simulink model "gm_sampleModel1982_sub"  (R2023a)
settings: Solver=VariableStepAuto  StartTime=0.0  StopTime=10.0  RelTol=1e-3
libraries: hdlsllib x1, simulink x1
settings Model: Creator=user1  LastModifiedBy=user1
settings OptimizationCC: BlockReduction=off  ConditionallyExecuteInputs=off
settings DebuggingCC: InheritedTsInSrcMsg=none

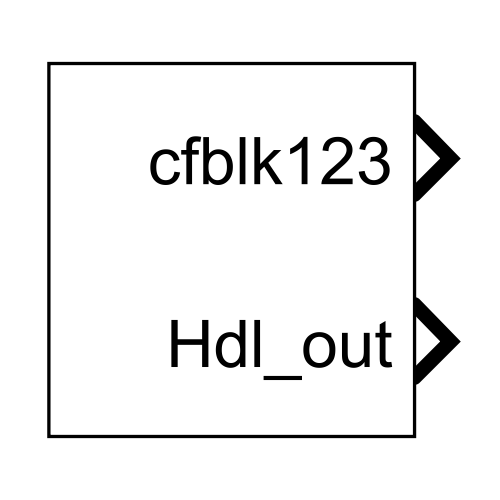
[thumbnail: Simulink's stored preview of the top-level diagram]
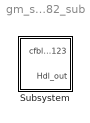
== system gm_sampleModel1982_sub ==
  Subsystem : Subsystem

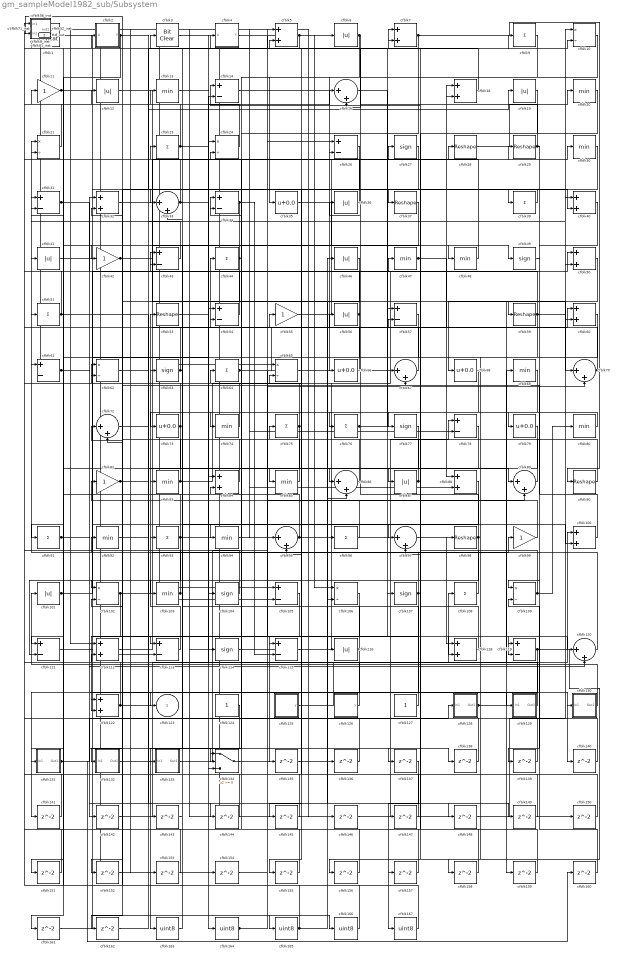
== system gm_sampleModel1982_sub/Subsystem ==
  cfblk1 : hdlsllib/Logic and Bit Operations/Bit Concat  numInputs=2
  cfblk{10,21,24,62,65,102,106,109} (8 alike) : Product  Inputs=*/  OutDataTypeStr=uint8  RndMeth=Zero  SaturateOnIntegerOverflow=on
  cfblk{5,7,18,32,40,50,60,84,88,100,112,118,122} (13 alike) : Sum  OutDataTypeStr=uint8
  cfblk{6,12,19,36,41,46,56,87,101,116} (10 alike) : Abs  OutDataTypeStr=uint8  SaturateOnIntegerOverflow=off
  cfblk{13,20,30,47..48,69,74,80,83,85,92,94,103} (13 alike) : MinMax  OutDataTypeStr=uint8
  cfblk{27,49,63,77,104,107,114} (7 alike) : Signum
  cfblk{14,26,31,34,43,54,57,61,78,105,111,113,115,119} (14 alike) : Sum  Inputs=+-  OutDataTypeStr=uint8
  cfblk{9,23,39,44,51,64,75..76,91,93,96,108} (12 alike) : Sum  Inputs=+  OutDataTypeStr=uint8
  cfblk{11,42,55,82,99} (5 alike) : Gain  OutDataTypeStr=uint8
  cfblk110_inst : Subsystem
  cfblk117_inst : Subsystem
  cfblk{16,33,67,70,72,86,89,95,97,120} (10 alike) : Sum  Inputs=|++  OutDataTypeStr=uint8
  cfblk121_inst : Subsystem
  cfblk124 : Constant  OutDataTypeStr=uint8  SampleTime=-1
  cfblk125 : Subsystem  mask(Counter Free-Running){NumBits=double(16), tsamp=double(-1)}
      mask prompts: NumBits "Simulink:masks:NumberOfBits_MP"; tsamp "Simulink:masks:SampleTime_MP"
      mask help: Simulink:masks:CounterFreeRunning_MD
  cfblk126 : Subsystem  mask(Counter Limited){uplimit=double(7), tsamp=double(-1)}
      mask prompts: uplimit "Simulink:masks:UpperLimit_MP"; tsamp "Simulink:masks:SampleTime_MP"
      mask help: Simulink:masks:CounterLimited_MD
      mask init:
      | nbits = double(8);
      | tsamp = double(-1);
      | uplimit = double(7);
  cfblk127 : Constant  OutDataTypeStr=uint8  SampleTime=-1
  cfblk128 : Subsystem
  cfblk129 : Subsystem
  cfblk130 : Subsystem
  cfblk131 : Subsystem
  cfblk132 : Subsystem
  cfblk133 : Subsystem
  cfblk134 : Switch  OutDataTypeStr=uint8  SaturateOnIntegerOverflow=off  InputSameDT=off
  cfblk{135..162} (28 alike) : Delay  SampleTime=1
  cfblk15_inst : Subsystem
  cfblk{163..167} (5 alike) : DataTypeConversion  OutDataTypeStr=uint8  SaturateOnIntegerOverflow=off  RndMeth=Floor
  cfblk17_inst : Subsystem
  cfblk2 : Subsystem  mask(Detect Fall Nonpositive){vinit=double(0), InputProcessing=Elements as channels (sample based), OutDataTypeStr=uint8}
      mask prompts: vinit "Simulink:masks:InitialCondition_MP"; InputProcessing "Simulink:masks:InputProcessing_MP"; OutDataTypeStr "Simulink:masks:OutputDataType_MP"
      mask help: Simulink:masks:DetectFallNonpositive_MD
      mask init:
      | InputProcessing = 'Elements as channels (sample based)';
      | OutDataTypeStr = 'uint8';
      | vinit = double(0);
      mask TypeOptions InputProcessing: Simulink:masks:ColumnsAsChannelsFrameBased | Simulink:masks:ElementsAsChannelsSampleBased
      mask TypeOptions OutDataTypeStr: Simulink:masks:uint8 | Simulink:masks:boolean
      mask Display: fprintf('U <= 0\n&  NOT\nU/z <= 0')
  cfblk22_inst : Subsystem
  cfblk25_inst : Subsystem
  cfblk{28..29,37,53,59,90,98} (7 alike) : Reshape
  cfblk3 : simulink/Logic and Bit Operations/Bit Clear  iBit=0
      settings: LibrarySourceBlock=|
      | hdlsllib/Logic and Bit
      | Operations/Bit Clear
  cfblk{35,66,68,73,79} (5 alike) : Bias  Bias=0.0  SaturateOnIntegerOverflow=off
  cfblk38_inst : Subsystem
  cfblk4 : Subsystem  mask(Detect Fall Nonpositive){vinit=double(0), InputProcessing=Elements as channels (sample based), OutDataTypeStr=uint8}
      mask prompts: vinit "Simulink:masks:InitialCondition_MP"; InputProcessing "Simulink:masks:InputProcessing_MP"; OutDataTypeStr "Simulink:masks:OutputDataType_MP"
      mask help: Simulink:masks:DetectFallNonpositive_MD
      mask init:
      | InputProcessing = 'Elements as channels (sample based)';
      | OutDataTypeStr = 'uint8';
      | vinit = double(0);
      mask TypeOptions InputProcessing: Simulink:masks:ColumnsAsChannelsFrameBased | Simulink:masks:ElementsAsChannelsSampleBased
      mask TypeOptions OutDataTypeStr: Simulink:masks:uint8 | Simulink:masks:boolean
      mask Display: fprintf('U <= 0\n&  NOT\nU/z <= 0')
  cfblk45_inst : Subsystem
  cfblk52_inst : Subsystem
  cfblk58_inst : Subsystem
  cfblk71_inst : Subsystem
  cfblk81_inst : Subsystem
  cfblk8_inst : Subsystem
  cfblk123 : Outport  OutDataTypeStr=uint8  SampleTime=1  VectorParamsAs1DForOutWhenUnconnected=off
  Hdl_out : Outport  Port=2  OutDataTypeStr=uint8
  wires:
  cfblk1/1 -> cfblk165/1
  cfblk10/1 -> cfblk66/1
  cfblk100/1 -> cfblk121_inst/2(in2)
  cfblk101/1 -> cfblk119/2, cfblk47/1
  cfblk102/1 -> cfblk28/1, cfblk27/1, cfblk122/2, cfblk99/1
  cfblk103/1 -> cfblk53/1, cfblk17_inst/1(in1)
  cfblk104/1 -> cfblk21/1
  cfblk105/1 -> cfblk122/1
  cfblk106/1 -> cfblk135/1
  cfblk107/1 -> cfblk61/1, cfblk115/1, cfblk132/1(In1)
  cfblk108/1 -> cfblk14/1
  cfblk109/1 -> cfblk55/1, cfblk80/1
  cfblk11/1 -> cfblk39/1, cfblk94/1
  cfblk110_inst/1(out1) -> cfblk113/2, cfblk105/1
  cfblk111/1 -> cfblk140/1
  cfblk112/1 -> cfblk44/1
  cfblk113/1 -> cfblk93/1
  cfblk114/1 -> cfblk30/1
  cfblk115/1 -> cfblk10/1
  cfblk116/1 -> cfblk63/1, cfblk141/1
  cfblk117_inst/1(out1) -> cfblk61/2, cfblk136/1
  cfblk118/1 -> cfblk7/1
  cfblk119/1 -> cfblk156/1, cfblk155/1
  cfblk12/1 -> cfblk129/1(In1)
  cfblk120/1 -> cfblk92/1
  cfblk121_inst/1(out1) -> cfblk116/1
  cfblk122/1 -> cfblk14/2, cfblk21/2, cfblk69/1
  cfblk124/1 -> cfblk163/1
  cfblk125/1(y) -> cfblk100/1
  cfblk126/1(y) -> cfblk64/1
  cfblk127/1 -> cfblk83/1
  cfblk128/1(Out1) -> cfblk159/1, cfblk130/1(In1)
  cfblk129/1(Out1) -> cfblk38_inst/1(in1)
  cfblk13/1 -> cfblk120/1
  cfblk130/1(Out1) -> cfblk101/1
  cfblk131/1(Out1) -> cfblk160/1, cfblk128/1(In1)
  cfblk132/1(Out1) -> cfblk108/1
  cfblk133/1(Out1) -> cfblk5/1
  cfblk134/1 -> cfblk50/1
  cfblk135/1 -> cfblk65/2
  cfblk136/1 -> cfblk112/2
  cfblk137/1 -> cfblk167/1
  cfblk138/1 -> cfblk45_inst/1(in1)
  cfblk139/1 -> cfblk62/1
  cfblk14/1 -> cfblk26/2
  cfblk140/1 -> cfblk52_inst/1(in1)
  cfblk141/1 -> cfblk81_inst/1(in1)
  cfblk142/1 -> cfblk86/2
  cfblk143/1 -> cfblk33/2
  cfblk144/1 -> cfblk43/1
  cfblk145/1 -> cfblk54/2
  cfblk146/1 -> cfblk78/1
  cfblk147/1 -> cfblk84/2
  cfblk148/1 -> cfblk50/2
  cfblk149/1 -> cfblk5/2
  cfblk15_inst/1(out1) -> cfblk110_inst/1(in1)
  cfblk150/1 -> cfblk17_inst/2(in2)
  cfblk151/1 -> cfblk22_inst/2(in2)
  cfblk152/1 -> cfblk102/2
  cfblk153/1 -> cfblk32/2
  cfblk154/1 -> cfblk89/2
  cfblk155/1 -> cfblk8_inst/2(in2)
  cfblk156/1 -> cfblk24/2
  cfblk157/1 -> cfblk34/1
  cfblk158/1 -> cfblk72/1
  cfblk159/1 -> cfblk97/2
  cfblk16/1 -> cfblk107/1
  cfblk160/1 -> cfblk109/2
  cfblk161/1 -> cfblk166/1
  cfblk162/1 -> cfblk7/2
  cfblk163/1 -> cfblk3/1
  cfblk164/1 -> cfblk70/2, cfblk67/2
  cfblk165/1 -> cfblk60/1, cfblk62/2
  cfblk166/1 -> cfblk1/1
  cfblk167/1 -> cfblk1/2
  cfblk17_inst/1(out1) -> cfblk67/1
  cfblk18/1 -> cfblk4/1(U)
  cfblk19/1 -> cfblk97/1
  cfblk2/1(Y) -> cfblk40/2, cfblk91/1
  cfblk20/1 -> cfblk77/1
  cfblk21/1 -> cfblk117_inst/1(in1)
  cfblk22_inst/1(out1) -> cfblk88/2, cfblk105/2, cfblk150/1
  cfblk23/1 -> cfblk59/1, cfblk12/1
  cfblk24/1 -> cfblk81_inst/2(in2)
  cfblk25_inst/1(out1) -> cfblk98/1, cfblk153/1
  cfblk26/1 -> cfblk145/1
  cfblk27/1 -> cfblk37/1
  cfblk28/1 -> cfblk20/1
  cfblk29/1 -> cfblk79/1, cfblk58_inst/1(in1)
  cfblk3/1 -> cfblk164/1
  cfblk30/1 -> cfblk72/2
  cfblk31/1 -> cfblk144/1, cfblk143/1
  cfblk32/1 -> cfblk48/1
  cfblk33/1 -> cfblk45_inst/2(in2), cfblk16/1
  cfblk34/1 -> cfblk73/1, cfblk115/2
  cfblk35/1 -> cfblk49/1
  cfblk36/1 -> cfblk15_inst/1(in1)
  cfblk37/1 -> cfblk161/1
  cfblk38_inst/1(out1) -> cfblk25_inst/2(in2), cfblk154/1
  cfblk39/1 -> cfblk33/1
  cfblk4/1(Y) -> cfblk10/2
  cfblk40/1 -> cfblk139/1
  cfblk41/1 -> cfblk114/1
  cfblk42/1 -> cfblk88/1, cfblk134/3, cfblk96/1
  cfblk43/1 -> cfblk31/1
  cfblk44/1 -> cfblk42/1, cfblk162/1
  cfblk45_inst/1(out1) -> cfblk78/2
  cfblk46/1 -> cfblk133/1(In1)
  cfblk47/1 -> cfblk60/2, cfblk157/1
  cfblk48/1 -> cfblk23/1
  cfblk49/1 -> cfblk109/1
  cfblk5/1 -> cfblk52_inst/2(in2), cfblk106/1
  cfblk50/1 -> cfblk68/1
  cfblk51/1 -> cfblk71_inst/2(in2), cfblk148/1
  cfblk52_inst/1(out1) -> cfblk112/1
  cfblk53/1 -> cfblk104/1
  cfblk54/1 -> cfblk32/1
  cfblk55/1 -> cfblk29/1
  cfblk56/1 -> cfblk22_inst/1(in1), cfblk106/2
  cfblk57/1 -> cfblk151/1
  cfblk58_inst/1(out1) -> cfblk95/1
  cfblk59/1 -> cfblk70/1, cfblk38_inst/2(in2), cfblk111/1
  cfblk6/1 -> cfblk35/1, cfblk16/2, cfblk117_inst/2(in2)
  cfblk60/1 -> cfblk158/1
  cfblk61/1 -> cfblk120/2, cfblk137/1
  cfblk62/1 -> cfblk19/1
  cfblk63/1 -> cfblk43/2, cfblk2/1(U)
  cfblk64/1 -> cfblk18/2, cfblk118/2
  cfblk65/1 -> cfblk46/1
  cfblk66/1 -> cfblk56/1
  cfblk67/1 -> cfblk24/1
  cfblk68/1 -> cfblk103/1
  cfblk69/1 -> cfblk95/2
  cfblk7/1 -> cfblk90/1, cfblk134/2
  cfblk70/1 -> cfblk18/1, cfblk121_inst/1(in1)
  cfblk71_inst/1(out1) -> cfblk147/1, cfblk146/1
  cfblk72/1 -> cfblk86/1
  cfblk73/1 -> cfblk110_inst/2(in2), cfblk131/1(In1)
  cfblk74/1 -> cfblk15_inst/2(in2)
  cfblk75/1 -> cfblk58_inst/2(in2), cfblk102/1
  cfblk76/1 -> cfblk57/1, cfblk119/1
  cfblk77/1 -> cfblk85/1
  cfblk78/1 -> cfblk134/1
  cfblk79/1 -> cfblk87/1
  cfblk8_inst/1(out1) -> cfblk65/1
  cfblk80/1 -> cfblk76/1
  cfblk81_inst/1(out1) -> cfblk6/1
  cfblk82/1 -> cfblk89/1, cfblk40/1
  cfblk83/1 -> cfblk25_inst/1(in1), cfblk100/2, cfblk9/1
  cfblk84/1 -> cfblk11/1
  cfblk85/1 -> cfblk34/2
  cfblk86/1 -> cfblk75/1
  cfblk87/1 -> cfblk41/1, cfblk13/1
  cfblk88/1 -> cfblk113/1
  cfblk89/1 -> cfblk54/1
  cfblk9/1 -> cfblk74/1
  cfblk90/1 -> cfblk8_inst/1(in1)
  cfblk91/1 -> cfblk142/1, cfblk123/1
  cfblk92/1 -> cfblk138/1
  cfblk93/1 -> cfblk57/2, cfblk31/2, cfblk111/2
  cfblk94/1 -> cfblk26/1
  cfblk95/1 -> cfblk149/1, cfblk51/1
  cfblk96/1 -> cfblk84/1
  cfblk97/1 -> cfblk118/1
  cfblk98/1 -> cfblk71_inst/1(in1), cfblk36/1, cfblk152/1
  cfblk99/1 -> cfblk82/1

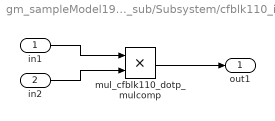
== system gm_sampleModel1982_sub/Subsystem/cfblk110_inst ==
  in1 : Inport  OutDataTypeStr=uint8  SampleTime=1
  in2 : Inport  Port=2  OutDataTypeStr=uint8  SampleTime=1
  mul_cfblk110_dotp_mulcomp : Product  Inputs=**  OutDataTypeStr=uint8  SampleTime=1
  out1 : Outport  OutDataTypeStr=uint8  SampleTime=1
  wires:
  in1/1 -> mul_cfblk110_dotp_mulcomp/1
  in2/1 -> mul_cfblk110_dotp_mulcomp/2
  mul_cfblk110_dotp_mulcomp/1 -> out1/1

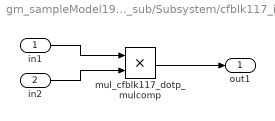
== system gm_sampleModel1982_sub/Subsystem/cfblk117_inst ==
  in1 : Inport  OutDataTypeStr=uint8  SampleTime=1
  in2 : Inport  Port=2  OutDataTypeStr=uint8  SampleTime=1
  mul_cfblk117_dotp_mulcomp : Product  Inputs=**  OutDataTypeStr=uint8  SampleTime=1
  out1 : Outport  OutDataTypeStr=uint8  SampleTime=1
  wires:
  in1/1 -> mul_cfblk117_dotp_mulcomp/1
  in2/1 -> mul_cfblk117_dotp_mulcomp/2
  mul_cfblk117_dotp_mulcomp/1 -> out1/1

== system gm_sampleModel1982_sub/Subsystem/cfblk121_inst ==
  in1 : Inport  OutDataTypeStr=uint8  SampleTime=1
  in2 : Inport  Port=2  OutDataTypeStr=uint8  SampleTime=1
  mul_cfblk121_dotp_mulcomp : Product  Inputs=**  OutDataTypeStr=uint8  SampleTime=1
  out1 : Outport  OutDataTypeStr=uint8  SampleTime=1
  wires:
  in1/1 -> mul_cfblk121_dotp_mulcomp/1
  in2/1 -> mul_cfblk121_dotp_mulcomp/2
  mul_cfblk121_dotp_mulcomp/1 -> out1/1

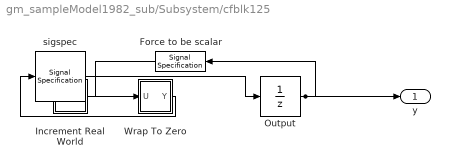
== system gm_sampleModel1982_sub/Subsystem/cfblk125 ==
  Force to be scalar : SignalSpecification  DisableCoverage=on  Dimensions=1
  Increment Real World : Subsystem  mask(Real World Value Increment){}
      mask help: Simulink:masks:RealWorldValueIncrement_MD
      mask Display: disp('V++')
  Output : UnitDelay  InitialCondition=0.0  SampleTime=tsamp  HasFrameUpgradeWarning=on
  Wrap To Zero : Subsystem  mask(Wrap To Zero){Threshold=double(65535)}
      mask prompts: Threshold "Simulink:masks:Threshold_MP"
      mask help: Simulink:masks:WrapToZero_MD
  sigspec : SignalSpecification  OutDataTypeStr=uint16  Dimensions=1
  y : Outport  SampleTime=1
  wires:
  Force to be scalar/1 -> Increment Real World/1(u)
  Increment Real World/1(y) -> Wrap To Zero/1(U)
  Output/1 -> Force to be scalar/1, y/1
  Wrap To Zero/1(Y) -> sigspec/1
  sigspec/1 -> Output/1

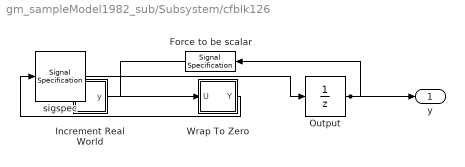
== system gm_sampleModel1982_sub/Subsystem/cfblk126 ==
  Force to be scalar : SignalSpecification  DisableCoverage=on  Dimensions=1
  Increment Real World : Subsystem  mask(Real World Value Increment){}
      mask help: Simulink:masks:RealWorldValueIncrement_MD
      mask Display: disp('V++')
  Output : UnitDelay  InitialCondition=0.0  SampleTime=tsamp  HasFrameUpgradeWarning=on
  Wrap To Zero : Subsystem  mask(Wrap To Zero){Threshold=double(7)}
      mask prompts: Threshold "Simulink:masks:Threshold_MP"
      mask help: Simulink:masks:WrapToZero_MD
  sigspec : SignalSpecification  OutDataTypeStr=uint8  Dimensions=1
  y : Outport  SampleTime=1
  wires:
  Force to be scalar/1 -> Increment Real World/1(u)
  Increment Real World/1(y) -> Wrap To Zero/1(U)
  Output/1 -> Force to be scalar/1, y/1
  Wrap To Zero/1(Y) -> sigspec/1
  sigspec/1 -> Output/1

== system gm_sampleModel1982_sub/Subsystem/cfblk128 ==
  In1 : Inport  OutDataTypeStr=uint8  PortDimensions=1  SampleTime=1
  Out1 : Outport  SampleTime=1
  wires:
  In1/1 -> Out1/1

== system gm_sampleModel1982_sub/Subsystem/cfblk129 ==
  In1 : Inport  OutDataTypeStr=uint8  PortDimensions=1  SampleTime=1
  Out1 : Outport  SampleTime=1
  wires:
  In1/1 -> Out1/1

== system gm_sampleModel1982_sub/Subsystem/cfblk130 ==
  In1 : Inport  OutDataTypeStr=uint8  PortDimensions=1  SampleTime=1
  Out1 : Outport  SampleTime=1
  wires:
  In1/1 -> Out1/1

== system gm_sampleModel1982_sub/Subsystem/cfblk131 ==
  In1 : Inport  OutDataTypeStr=uint8  PortDimensions=1  SampleTime=1
  Out1 : Outport  SampleTime=1
  wires:
  In1/1 -> Out1/1

== system gm_sampleModel1982_sub/Subsystem/cfblk132 ==
  In1 : Inport  OutDataTypeStr=uint8  PortDimensions=1  SampleTime=1
  Out1 : Outport  SampleTime=1
  wires:
  In1/1 -> Out1/1

== system gm_sampleModel1982_sub/Subsystem/cfblk133 ==
  In1 : Inport  OutDataTypeStr=uint8  PortDimensions=1  SampleTime=1
  Out1 : Outport  SampleTime=1
  wires:
  In1/1 -> Out1/1

== system gm_sampleModel1982_sub/Subsystem/cfblk15_inst ==
  in1 : Inport  OutDataTypeStr=uint8  SampleTime=1
  in2 : Inport  Port=2  OutDataTypeStr=uint8  SampleTime=1
  mul_cfblk15_dotp_mulcomp : Product  Inputs=**  OutDataTypeStr=uint8  SampleTime=1
  out1 : Outport  OutDataTypeStr=uint8  SampleTime=1
  wires:
  in1/1 -> mul_cfblk15_dotp_mulcomp/1
  in2/1 -> mul_cfblk15_dotp_mulcomp/2
  mul_cfblk15_dotp_mulcomp/1 -> out1/1

== system gm_sampleModel1982_sub/Subsystem/cfblk17_inst ==
  in1 : Inport  OutDataTypeStr=uint8  SampleTime=1
  in2 : Inport  Port=2  OutDataTypeStr=uint8  SampleTime=1
  mul_cfblk17_dotp_mulcomp : Product  Inputs=**  OutDataTypeStr=uint8  SampleTime=1
  out1 : Outport  OutDataTypeStr=uint8  SampleTime=1
  wires:
  in1/1 -> mul_cfblk17_dotp_mulcomp/1
  in2/1 -> mul_cfblk17_dotp_mulcomp/2
  mul_cfblk17_dotp_mulcomp/1 -> out1/1

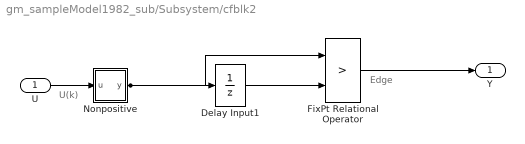
== system gm_sampleModel1982_sub/Subsystem/cfblk2 ==
  note: U(k)
  note: Edge
  U : Inport  OutDataTypeStr=uint8  SampleTime=1
  Delay Input1 : UnitDelay  Description=Store in Global RAM  DisableCoverage=on  InitialCondition=vinit  SampleTime=-1  HasFrameUpgradeWarning=on
  FixPt Relational Operator : RelationalOperator  Operator=>  OutDataTypeStr=fixdt(0, 8)  ZeroCross=off  InputSameDT=off
  Nonpositive : Subsystem  mask(Compare To Zero){relop=<=, OutDataTypeStr=boolean, ZeroCross=off}
      mask prompts: relop "Simulink:masks:Operator_MP"; OutDataTypeStr "Simulink:masks:OutputDataType_MP"; ZeroCross "Simulink:masks:EnableZerocrossingDetection_MP"
      mask help: Simulink:masks:CompareToZero_MD
      mask init:
      | OutDataTypeStr = 'boolean';
      | ZeroCross = 'off';
      | blkName = 'sampleModel1982_sub/Subsystem/cfblk2/Nonpositive';
      | relop = '<=';
      | setValue = 'boolean';
      mask TypeOptions relop: == | ~= | < | <= | >= | >
      mask TypeOptions OutDataTypeStr: Simulink:masks:uint8 | Simulink:masks:boolean
      mask Callback ZeroCross: sl('zeroCrossEnable', gcbh);
      mask Display: disp([relop,' 0'])
  Y : Outport  SampleTime=1
  wires:
  U/1 -> Nonpositive/1(u)
  Delay Input1/1 -> FixPt Relational Operator/2
  FixPt Relational Operator/1 -> Y/1
  Nonpositive/1(y) -> FixPt Relational Operator/1, Delay Input1/1

== system gm_sampleModel1982_sub/Subsystem/cfblk22_inst ==
  in1 : Inport  OutDataTypeStr=uint8  SampleTime=1
  in2 : Inport  Port=2  OutDataTypeStr=uint8  SampleTime=1
  mul_cfblk22_dotp_mulcomp : Product  Inputs=**  OutDataTypeStr=uint8  SampleTime=1
  out1 : Outport  OutDataTypeStr=uint8  SampleTime=1
  wires:
  in1/1 -> mul_cfblk22_dotp_mulcomp/1
  in2/1 -> mul_cfblk22_dotp_mulcomp/2
  mul_cfblk22_dotp_mulcomp/1 -> out1/1

== system gm_sampleModel1982_sub/Subsystem/cfblk25_inst ==
  in1 : Inport  OutDataTypeStr=uint8  SampleTime=1
  in2 : Inport  Port=2  OutDataTypeStr=uint8  SampleTime=1
  mul_cfblk25_dotp_mulcomp : Product  Inputs=**  OutDataTypeStr=uint8  SampleTime=1
  out1 : Outport  OutDataTypeStr=uint8  SampleTime=1
  wires:
  in1/1 -> mul_cfblk25_dotp_mulcomp/1
  in2/1 -> mul_cfblk25_dotp_mulcomp/2
  mul_cfblk25_dotp_mulcomp/1 -> out1/1

== system gm_sampleModel1982_sub/Subsystem/cfblk38_inst ==
  in1 : Inport  OutDataTypeStr=uint8  SampleTime=1
  in2 : Inport  Port=2  OutDataTypeStr=uint8  SampleTime=1
  mul_cfblk38_dotp_mulcomp : Product  Inputs=**  OutDataTypeStr=uint8  SampleTime=1
  out1 : Outport  OutDataTypeStr=uint8  SampleTime=1
  wires:
  in1/1 -> mul_cfblk38_dotp_mulcomp/1
  in2/1 -> mul_cfblk38_dotp_mulcomp/2
  mul_cfblk38_dotp_mulcomp/1 -> out1/1

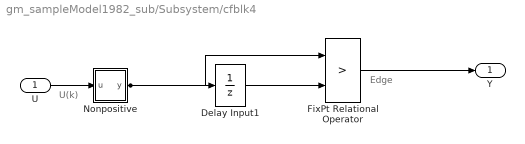
== system gm_sampleModel1982_sub/Subsystem/cfblk4 ==
  note: U(k)
  note: Edge
  U : Inport  OutDataTypeStr=uint8  SampleTime=1
  Delay Input1 : UnitDelay  Description=Store in Global RAM  DisableCoverage=on  InitialCondition=vinit  SampleTime=-1  HasFrameUpgradeWarning=on
  FixPt Relational Operator : RelationalOperator  Operator=>  OutDataTypeStr=fixdt(0, 8)  ZeroCross=off  InputSameDT=off
  Nonpositive : Subsystem  mask(Compare To Zero){relop=<=, OutDataTypeStr=boolean, ZeroCross=off}
      mask prompts: relop "Simulink:masks:Operator_MP"; OutDataTypeStr "Simulink:masks:OutputDataType_MP"; ZeroCross "Simulink:masks:EnableZerocrossingDetection_MP"
      mask help: Simulink:masks:CompareToZero_MD
      mask init:
      | OutDataTypeStr = 'boolean';
      | ZeroCross = 'off';
      | blkName = 'sampleModel1982_sub/Subsystem/cfblk4/Nonpositive';
      | relop = '<=';
      | setValue = 'boolean';
      mask TypeOptions relop: == | ~= | < | <= | >= | >
      mask TypeOptions OutDataTypeStr: Simulink:masks:uint8 | Simulink:masks:boolean
      mask Callback ZeroCross: sl('zeroCrossEnable', gcbh);
      mask Display: disp([relop,' 0'])
  Y : Outport  SampleTime=1
  wires:
  U/1 -> Nonpositive/1(u)
  Delay Input1/1 -> FixPt Relational Operator/2
  FixPt Relational Operator/1 -> Y/1
  Nonpositive/1(y) -> FixPt Relational Operator/1, Delay Input1/1

== system gm_sampleModel1982_sub/Subsystem/cfblk45_inst ==
  in1 : Inport  OutDataTypeStr=uint8  SampleTime=1
  in2 : Inport  Port=2  OutDataTypeStr=uint8  SampleTime=1
  mul_cfblk45_dotp_mulcomp : Product  Inputs=**  OutDataTypeStr=uint8  SampleTime=1
  out1 : Outport  OutDataTypeStr=uint8  SampleTime=1
  wires:
  in1/1 -> mul_cfblk45_dotp_mulcomp/1
  in2/1 -> mul_cfblk45_dotp_mulcomp/2
  mul_cfblk45_dotp_mulcomp/1 -> out1/1

== system gm_sampleModel1982_sub/Subsystem/cfblk52_inst ==
  in1 : Inport  OutDataTypeStr=uint8  SampleTime=1
  in2 : Inport  Port=2  OutDataTypeStr=uint8  SampleTime=1
  mul_cfblk52_dotp_mulcomp : Product  Inputs=**  OutDataTypeStr=uint8  SampleTime=1
  out1 : Outport  OutDataTypeStr=uint8  SampleTime=1
  wires:
  in1/1 -> mul_cfblk52_dotp_mulcomp/1
  in2/1 -> mul_cfblk52_dotp_mulcomp/2
  mul_cfblk52_dotp_mulcomp/1 -> out1/1

== system gm_sampleModel1982_sub/Subsystem/cfblk58_inst ==
  in1 : Inport  OutDataTypeStr=uint8  SampleTime=1
  in2 : Inport  Port=2  OutDataTypeStr=uint8  SampleTime=1
  mul_cfblk58_dotp_mulcomp : Product  Inputs=**  OutDataTypeStr=uint8  SampleTime=1
  out1 : Outport  OutDataTypeStr=uint8  SampleTime=1
  wires:
  in1/1 -> mul_cfblk58_dotp_mulcomp/1
  in2/1 -> mul_cfblk58_dotp_mulcomp/2
  mul_cfblk58_dotp_mulcomp/1 -> out1/1

== system gm_sampleModel1982_sub/Subsystem/cfblk71_inst ==
  in1 : Inport  OutDataTypeStr=uint8  SampleTime=1
  in2 : Inport  Port=2  OutDataTypeStr=uint8  SampleTime=1
  mul_cfblk71_dotp_mulcomp : Product  Inputs=**  OutDataTypeStr=uint8  SampleTime=1
  out1 : Outport  OutDataTypeStr=uint8  SampleTime=1
  wires:
  in1/1 -> mul_cfblk71_dotp_mulcomp/1
  in2/1 -> mul_cfblk71_dotp_mulcomp/2
  mul_cfblk71_dotp_mulcomp/1 -> out1/1

== system gm_sampleModel1982_sub/Subsystem/cfblk81_inst ==
  in1 : Inport  OutDataTypeStr=uint8  SampleTime=1
  in2 : Inport  Port=2  OutDataTypeStr=uint8  SampleTime=1
  mul_cfblk81_dotp_mulcomp : Product  Inputs=**  OutDataTypeStr=uint8  SampleTime=1
  out1 : Outport  OutDataTypeStr=uint8  SampleTime=1
  wires:
  in1/1 -> mul_cfblk81_dotp_mulcomp/1
  in2/1 -> mul_cfblk81_dotp_mulcomp/2
  mul_cfblk81_dotp_mulcomp/1 -> out1/1

== system gm_sampleModel1982_sub/Subsystem/cfblk8_inst ==
  in1 : Inport  OutDataTypeStr=uint8  SampleTime=1
  in2 : Inport  Port=2  OutDataTypeStr=uint8  SampleTime=1
  mul_cfblk8_dotp_mulcomp : Product  Inputs=**  OutDataTypeStr=uint8  SampleTime=1
  out1 : Outport  OutDataTypeStr=uint8  SampleTime=1
  wires:
  in1/1 -> mul_cfblk8_dotp_mulcomp/1
  in2/1 -> mul_cfblk8_dotp_mulcomp/2
  mul_cfblk8_dotp_mulcomp/1 -> out1/1

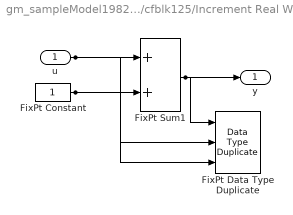
== system gm_sampleModel1982_sub/Subsystem/cfblk125/Increment Real World ==
  u : Inport  OutDataTypeStr=uint16  SampleTime=1
  FixPt Constant : Constant  DisableCoverage=on  OutDataTypeStr=Inherit: Inherit via back propagation  SampleTime=-1
  FixPt Data Type Duplicate : DataTypeDuplicate  DisableCoverage=on  NumInputPorts=3
  FixPt Sum1 : Sum  InputSameDT=on  OutDataTypeStr=Inherit: Inherit via back propagation  LockScale=on
  y : Outport  SampleTime=1
  wires:
  u/1 -> FixPt Sum1/1, FixPt Data Type Duplicate/2
  FixPt Constant/1 -> FixPt Sum1/2, FixPt Data Type Duplicate/3
  FixPt Sum1/1 -> FixPt Data Type Duplicate/1, y/1

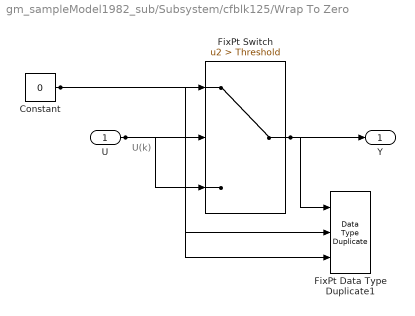
== system gm_sampleModel1982_sub/Subsystem/cfblk125/Wrap To Zero ==
  note: U(k)
  U : Inport  OutDataTypeStr=uint16  SampleTime=1
  Constant : Constant  DisableCoverage=on  Value=0  OutDataTypeStr=Inherit: Inherit via back propagation  SampleTime=-1
  FixPt Data Type Duplicate1 : DataTypeDuplicate  DisableCoverage=on  NumInputPorts=3
  FixPt Switch : Switch  Criteria=u2 > Threshold  Threshold=Threshold  OutDataTypeStr=Inherit: Inherit via back propagation  ZeroCross=off  SaturateOnIntegerOverflow=off  InputSameDT=off
  Y : Outport  SampleTime=1
  wires:
  U/1 -> FixPt Switch/3, FixPt Switch/2, FixPt Data Type Duplicate1/2
  Constant/1 -> FixPt Switch/1, FixPt Data Type Duplicate1/3
  FixPt Switch/1 -> FixPt Data Type Duplicate1/1, Y/1

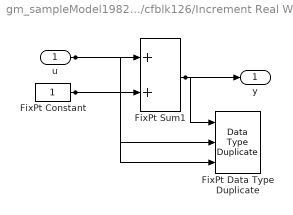
== system gm_sampleModel1982_sub/Subsystem/cfblk126/Increment Real World ==
  u : Inport  OutDataTypeStr=uint8  SampleTime=1
  FixPt Constant : Constant  DisableCoverage=on  OutDataTypeStr=Inherit: Inherit via back propagation  SampleTime=-1
  FixPt Data Type Duplicate : DataTypeDuplicate  DisableCoverage=on  NumInputPorts=3
  FixPt Sum1 : Sum  InputSameDT=on  OutDataTypeStr=Inherit: Inherit via back propagation  LockScale=on
  y : Outport  SampleTime=1
  wires:
  u/1 -> FixPt Sum1/1, FixPt Data Type Duplicate/2
  FixPt Constant/1 -> FixPt Sum1/2, FixPt Data Type Duplicate/3
  FixPt Sum1/1 -> FixPt Data Type Duplicate/1, y/1

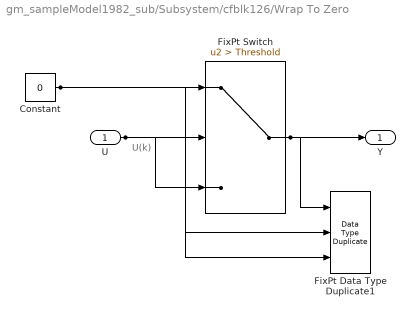
== system gm_sampleModel1982_sub/Subsystem/cfblk126/Wrap To Zero ==
  note: U(k)
  U : Inport  OutDataTypeStr=uint8  SampleTime=1
  Constant : Constant  DisableCoverage=on  Value=0  OutDataTypeStr=Inherit: Inherit via back propagation  SampleTime=-1
  FixPt Data Type Duplicate1 : DataTypeDuplicate  DisableCoverage=on  NumInputPorts=3
  FixPt Switch : Switch  Criteria=u2 > Threshold  Threshold=Threshold  OutDataTypeStr=Inherit: Inherit via back propagation  ZeroCross=off  SaturateOnIntegerOverflow=off  InputSameDT=off
  Y : Outport  SampleTime=1
  wires:
  U/1 -> FixPt Switch/3, FixPt Switch/2, FixPt Data Type Duplicate1/2
  Constant/1 -> FixPt Switch/1, FixPt Data Type Duplicate1/3
  FixPt Switch/1 -> FixPt Data Type Duplicate1/1, Y/1

== system gm_sampleModel1982_sub/Subsystem/cfblk2/Nonpositive ==
  u : Inport  OutDataTypeStr=uint8  SampleTime=1
  Compare : RelationalOperator  Operator=<=  OutDataTypeStr=boolean  ZeroCross=off
  Constant : Constant  DisableCoverage=on  Value=0  OutDataTypeStr=Inherit: Inherit via back propagation  SampleTime=-1  PreserveConstantTs=on
  y : Outport  SampleTime=1
  wires:
  u/1 -> Compare/1
  Compare/1 -> y/1
  Constant/1 -> Compare/2

== system gm_sampleModel1982_sub/Subsystem/cfblk4/Nonpositive ==
  u : Inport  OutDataTypeStr=uint8  SampleTime=1
  Compare : RelationalOperator  Operator=<=  OutDataTypeStr=boolean  ZeroCross=off
  Constant : Constant  DisableCoverage=on  Value=0  OutDataTypeStr=Inherit: Inherit via back propagation  SampleTime=-1  PreserveConstantTs=on
  y : Outport  SampleTime=1
  wires:
  u/1 -> Compare/1
  Compare/1 -> y/1
  Constant/1 -> Compare/2
